simulink model "BPSK"  (Simulink 7.2)
settings: Solver=ode45  StartTime=0.0  StopTime=100  RelTol=1e-3
libraries: commrandsrc2 x1, dsparch4 x1
settings Model: Creator=usuario  LastModifiedBy=USUARIO
settings OptimizationCC: InitFltsAndDblsToZero=on
settings DebuggingCC: SaveWithParameterizedLinksMsg=none  SignalResolutionControl=TryResolveAllWithWarning  MultiTaskDSMMsg=warning  MultiTaskCondExecSysMsg=none
settings RTWCC: IncludeERTFirstTime=on
settings GRTTargetCC: TargetFcnLib=ansi_tfl_tmw.mat

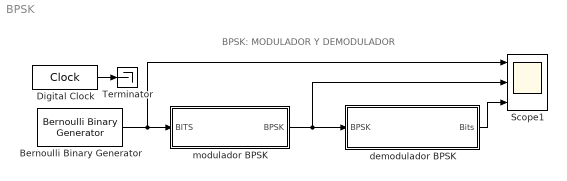
== system BPSK ==
  note: BPSK: MODULADOR Y DEMODULADOR
  Bernoulli Binary Generator : commrandsrc2/Bernoulli Binary Generator  DialogController=commDDGCreate  DialogControllerArgs=DataTag0  SystemSampleTime=-1  P=0.5  seed=51  Ts=5  frameBased=off  sampPerFrame=1  orient=off  outDataType=double
  Digital Clock : DigitalClock  SampleTime=0.001
  Scope1 : Scope  NumInputPorts=3
      settings: YMin=-5~-5~-5  YMax=5~5~5  SaveName=ScopeData3
  Terminator : Terminator
  demodulador BPSK : Subsystem
  modulador BPSK : Subsystem
  wires:
  Bernoulli Binary Generator/1 -> modulador BPSK/1(BITS), Scope1/1
  modulador BPSK/1(BPSK) -> demodulador BPSK/1(BPSK), Scope1/2
  demodulador BPSK/1(Bits) -> Scope1/3
  Digital Clock/1 -> Terminator/1

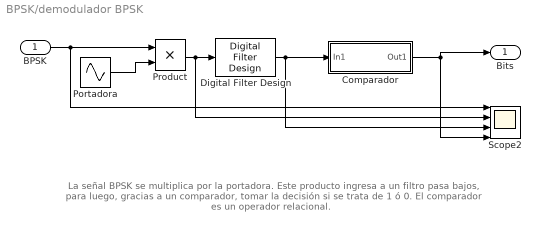
== system BPSK/demodulador BPSK ==
  note: La señal BPSK se multiplica por la portadora.
      | Este producto ingresa a un filtro
      | pasa bajos, para luego, gracias a un
      | comparador, tomar la decisión si se trata de
      | 1 ó 0. El comparador es un operador relacional.
  BPSK : Inport  OutDataType=sfix(16)  OutScaling=2^0
  Comparador : Subsystem
  Digital Filter Design : dsparch4/Digital Filter Design  SystemSampleTime=-1  mwdsp_browser_bugfix_var=off
  Portadora : Sin  SineType=Sample based  Frequency=2*10*pi  Samples=50  SampleTime=1/20
  Product : Product  OutDataType=sfix(16)  OutScaling=2^0  RndMeth=Zero
  Scope2 : Scope  NumInputPorts=4
      settings: YMin=-2~-3~-3~-5  YMax=2~3~3~5
  Bits : Outport  OutDataType=sfix(16)  OutScaling=2^0
  wires:
  BPSK/1 -> Scope2/1, Product/1
  Portadora/1 -> Product/2
  Product/1 -> Digital Filter Design/1, Scope2/2
  Digital Filter Design/1 -> Scope2/3, Comparador/1(In1)
  Comparador/1(Out1) -> Scope2/4, Bits/1

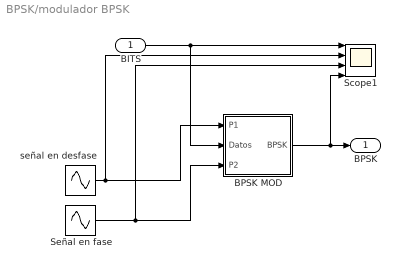
== system BPSK/modulador BPSK ==
  BITS : Inport  OutDataType=sfix(16)  OutScaling=2^0
  BPSK MOD : Subsystem
  Scope1 : Scope  NumInputPorts=4
      settings: YMin=-2~-3~-3~-3  YMax=2~3~3~3
  Señal en fase : Sin  SineType=Sample based  Frequency=2*10*pi  Phase=-pi  Samples=50  SampleTime=1/20  Offset=25
  señal en desfase : Sin  SineType=Sample based  Frequency=2*10*pi  Samples=50  SampleTime=1/20
  BPSK : Outport  OutDataType=sfix(16)  OutScaling=2^0
  wires:
  BITS/1 -> Scope1/1, BPSK MOD/2(Datos)
  señal en desfase/1 -> Scope1/2, BPSK MOD/1(P1)
  Señal en fase/1 -> Scope1/3, BPSK MOD/3(P2)
  BPSK MOD/1(BPSK) -> Scope1/4, BPSK/1

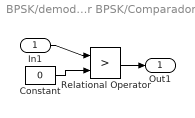
== system BPSK/demodulador BPSK/Comparador ==
  In1 : Inport  OutDataType=sfix(16)  OutScaling=2^0
  Constant : Constant  Value=0  OutDataType=sfix(16)  OutScaling=2^0
  Relational Operator : RelationalOperator  Operator=>  LogicOutDataTypeMode=boolean  OutDataTypeStr=boolean
  Out1 : Outport  OutDataType=sfix(16)  OutScaling=2^0
  wires:
  Constant/1 -> Relational Operator/2
  In1/1 -> Relational Operator/1
  Relational Operator/1 -> Out1/1

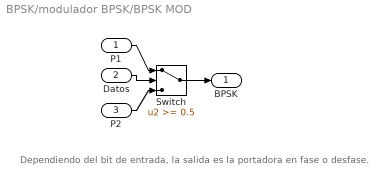
== system BPSK/modulador BPSK/BPSK MOD ==
  note: Dependiendo del bit
      | de entrada,
      | la salida es la portadora
      | en fase o desfase.
  P1 : Inport  OutDataType=sfix(16)  OutScaling=2^0
  Datos : Inport  Port=2  OutDataType=sfix(16)  OutScaling=2^0
  P2 : Inport  Port=3  OutDataType=sfix(16)  OutScaling=2^0
  Switch : Switch  Threshold=0.5
  BPSK : Outport  OutDataType=sfix(16)  OutScaling=2^0
  wires:
  P1/1 -> Switch/1
  Datos/1 -> Switch/2
  Switch/1 -> BPSK/1
  P2/1 -> Switch/3
